simulink library "halin"  (R2021b)
settings: Solver=VariableStepAuto  StartTime=0.0  StopTime=10.0  RelTol=1e-3
undefined symbols (not defined in the file): KHAL_CAN1ABM1E2E_flg, KHAL_CAN1EPB1E2E_flg, KHAL_CAN1EPS1E2E_flg, KHAL_CAN1ESC1E2E_flg, KHAL_CAN1ESC5E2E_flg, KHAL_CAN3BMS1E2E_flg, KHAL_CAN3BMS6E2E_flg, KHAL_CAN3CCU1E2E_flg, KHAL_CAN3CCU2E2E_flg, KHAL_CAN3MCUNF1E2E_flg, KHAL_CAN3MCUNR1E2E_flg, KHAL_CAN3Shifter1E2E_flg, KHAL_CAN3Shifter2E2E_flg, KHAL_CAN6FCM2E2E_flg, KHAL_CAN6FCM4E2E_flg, TRUE
libraries: simulink x645, FVT_lib x207, hcu_lib x59
(part 5 of 23)

== system halin/HAL_IN/CAN5 ==
  DT_CAN5_SG_TBOX1 : Inport
  DT_CAN5_SG_TBOX2 : Inport  Port=2
  DT_CAN5_SG_TBOX3 : Inport  Port=3
  UnitConverter{,2,4,8..10} (6 alike) : DataTypeConversion  OutDataTypeStr=uint8
  UnitConverter{1,6,11..27} (19 alike) : DataTypeConversion  OutDataTypeStr=single
  UnitConverter28 : DataTypeConversion  OutDataTypeStr=uint32
  UnitConverter29 : DataTypeConversion  OutDataTypeStr=uint32
  UnitConverter3 : DataTypeConversion  OutDataTypeStr=uint16
  UnitConverter5 : DataTypeConversion  OutDataTypeStr=boolean
  UnitConverter7 : DataTypeConversion  OutDataTypeStr=boolean
  VHAL_CANMsgInvalidTBOX1_flg : Subsystem  AncestorBlock=FVT_lib/hal/MsgTimeoutJudge_CAN_AUTOSAR
      mask help: MeasumentTrigerEvent
      mask Display: fprintf('MsgTimeoutJudge_CAN\nAUTOSAR');
  VHAL_CANMsgInvalidTBOX2_flg : Subsystem  AncestorBlock=FVT_lib/hal/MsgTimeoutJudge_CAN_AUTOSAR
      mask help: MeasumentTrigerEvent
      mask Display: fprintf('MsgTimeoutJudge_CAN\nAUTOSAR');
  VHAL_CANMsgInvalidTBOX3_flg : Subsystem  AncestorBlock=FVT_lib/hal/MsgTimeoutJudge_CAN_AUTOSAR
      mask help: MeasumentTrigerEvent
      mask Display: fprintf('MsgTimeoutJudge_CAN\nAUTOSAR');
  bus_creator : BusCreator  Inputs=33
  HAL_CAN5_outputs : Outport
  wires:
  DT_CAN5_SG_TBOX1/1 -> [DT_CAN5_SG_TBOX1]
  DT_CAN5_SG_TBOX2/1 -> [DT_CAN5_SG_TBOX2]
  DT_CAN5_SG_TBOX3/1 -> [DT_CAN5_SG_TBOX3]
  bus_creator/1 -> HAL_CAN5_outputs/1
  VHAL_CANMsgInvalidTBOX1_flg/1(Out) -> bus_creator/1
  UnitConverter/1 -> bus_creator/2  "VHAL_CbnPreACEnaReq_enum"
  [VHAL_CbnPreACEnaReq_enum] -> UnitConverter/1
  UnitConverter1/1 -> bus_creator/3  "VHAL_PowerOffTSet_cnt"
  [VHAL_PowerOffTSet_cnt] -> UnitConverter1/1
  UnitConverter2/1 -> bus_creator/4  "VHAL_ReOutsideMirror_enum"
  [VHAL_ReOutsideMirror_enum] -> UnitConverter2/1
  UnitConverter3/1 -> bus_creator/5  "VHAL_ReDoorLock_enum"
  [VHAL_ReDoorLock_enum] -> UnitConverter3/1
  UnitConverter4/1 -> bus_creator/6  "VHAL_RePwrReqTbox_enum"
  [VHAL_RePwrReqTbox_enum] -> UnitConverter4/1
  UnitConverter5/1 -> bus_creator/7  "VHAL_ReRadio_flg"
  [VHAL_ReRadio_flg] -> UnitConverter5/1
  UnitConverter6/1 -> bus_creator/8  "VHAL_RemoteACTemp_C"
  [VHAL_RemoteACTemp_C] -> UnitConverter6/1
  UnitConverter7/1 -> bus_creator/9  "VHAL_RemoteAutoReq_flg"
  [VHAL_RemoteAutoReq_flg] -> UnitConverter7/1
  UnitConverter8/1 -> bus_creator/10  "VHAL_TBOXNETSIGSTR_enum"
  [VHAL_TBOXNETSIGSTR_enum] -> UnitConverter8/1
  UnitConverter9/1 -> bus_creator/11  "VHAL_TBOXRemotePW_enum"
  [VHAL_TBOXRemotePW_enum] -> UnitConverter9/1
  UnitConverter10/1 -> bus_creator/12  "VHAL_TBOXTESTSTATUS_enum"
  [VHAL_TBOXTESTSTATUS_enum] -> UnitConverter10/1
  VHAL_CANMsgInvalidTBOX2_flg/1(Out) -> bus_creator/13
  UnitConverter11/1 -> bus_creator/14  "VHAL_TimeSyncFromBSDay_DAY"
  [VHAL_TimeSyncFromBSDay_DAY] -> UnitConverter11/1
  UnitConverter12/1 -> bus_creator/15  "VHAL_TimeSyncFromBSHour_hr"
  [VHAL_TimeSyncFromBSHour_hr] -> UnitConverter12/1
  UnitConverter13/1 -> bus_creator/16  "VHAL_TimeSyncFromBSMinute_min"
  [VHAL_TimeSyncFromBSMinute_min] -> UnitConverter13/1
  UnitConverter14/1 -> bus_creator/17  "VHAL_TimeSyncFromBSMonth_MONTH"
  [VHAL_TimeSyncFromBSMonth_MONTH] -> UnitConverter14/1
  UnitConverter15/1 -> bus_creator/18  "VHAL_TimeSyncFromBSSecond_s"
  [VHAL_TimeSyncFromBSSecond_s] -> UnitConverter15/1
  UnitConverter16/1 -> bus_creator/19  "VHAL_TimeSyncFromBSYear_YEAR"
  [VHAL_TimeSyncFromBSYear_YEAR] -> UnitConverter16/1
  VHAL_CANMsgInvalidTBOX3_flg/1(Out) -> bus_creator/20
  UnitConverter17/1 -> bus_creator/21  "VHAL_ChargePercentSet_pct"
  [VHAL_ChargePercentSet_pct] -> UnitConverter17/1
  UnitConverter18/1 -> bus_creator/22  "VHAL_ReserveChargeOFFDay_DAY"
  [VHAL_ReserveChargeOFFDay_DAY] -> UnitConverter18/1
  UnitConverter19/1 -> bus_creator/23  "VHAL_ReserveChargeOFFHour_hr"
  [VHAL_ReserveChargeOFFHour_hr] -> UnitConverter19/1
  UnitConverter20/1 -> bus_creator/24  "VHAL_ReserveChargeOFFMinute_min"
  [VHAL_ReserveChargeOFFMinute_min] -> UnitConverter20/1
  UnitConverter21/1 -> bus_creator/25  "VHAL_ReserveChargeOFFMonth_MONTH"
  [VHAL_ReserveChargeOFFMonth_MONTH] -> UnitConverter21/1
  UnitConverter22/1 -> bus_creator/26  "VHAL_ReserveChargeOFFYear_YEAR"
  [VHAL_ReserveChargeOFFYear_YEAR] -> UnitConverter22/1
  UnitConverter23/1 -> bus_creator/27  "VHAL_ReserveChargeOnDay_DAY"
  [VHAL_ReserveChargeOnDay_DAY] -> UnitConverter23/1
  UnitConverter24/1 -> bus_creator/28  "VHAL_ReserveChargeOnHour_hr"
  [VHAL_ReserveChargeOnHour_hr] -> UnitConverter24/1
  UnitConverter25/1 -> bus_creator/29  "VHAL_ReserveChargeOnMinute_min"
  [VHAL_ReserveChargeOnMinute_min] -> UnitConverter25/1
  UnitConverter26/1 -> bus_creator/30  "VHAL_ReserveChargeOnMonth_MONTH"
  [VHAL_ReserveChargeOnMonth_MONTH] -> UnitConverter26/1
  UnitConverter27/1 -> bus_creator/31  "VHAL_ReserveChargeOnYear_YEAR"
  [VHAL_ReserveChargeOnYear_YEAR] -> UnitConverter27/1
  UnitConverter28/1 -> bus_creator/32  "VHAL_TBOXHWVER_enum"
  [VHAL_TBOXHWVER_enum] -> UnitConverter28/1
  UnitConverter29/1 -> bus_creator/33  "VHAL_TBOXSWVER_enum"
  [VHAL_TBOXSWVER_enum] -> UnitConverter29/1

== system halin/HAL_IN/CAN6 ==
  DT_CAN6_SG_FCM1 : Inport
  DT_CAN6_SG_FCM2 : Inport  Port=2
  DT_CAN6_SG_FCM3 : Inport  Port=3
  DT_CAN6_SG_FCM4 : Inport  Port=4
  DT_CAN6_SG_SRR1 : Inport  Port=5
  FCM1 : Subsystem
  FCM2 : Subsystem
  FCM3 : Subsystem
  FCM4 : Subsystem
  SRR1 : Subsystem
  UnitConverter{,1..4,6..7,29..30,44,64..79,82..83,85..86} (30 alike) : DataTypeConversion  OutDataTypeStr=single
  UnitConverter{5,10..14,16,20,22..28,31..35,37..38,41..43,45,47,49,55,59..60,63,88..89,92..93} (36 alike) : DataTypeConversion  OutDataTypeStr=uint8
  UnitConverter{8..9,15,17..19,21,36,39..40,46,48,50..54,56..58,61..62,80..81,84,87,90..91} (28 alike) : DataTypeConversion  OutDataTypeStr=boolean
  VHAL_CANMsgInvalidFCM1_flg : Subsystem  AncestorBlock=FVT_lib/hal/MsgTimeoutJudge_CAN_AUTOSAR
      mask help: MeasumentTrigerEvent
      mask Display: fprintf('MsgTimeoutJudge_CAN\nAUTOSAR');
  VHAL_CANMsgInvalidFCM2_flg : Subsystem  AncestorBlock=FVT_lib/hal/MsgTimeoutJudge_CAN_AUTOSAR
      mask help: MeasumentTrigerEvent
      mask Display: fprintf('MsgTimeoutJudge_CAN\nAUTOSAR');
  VHAL_CANMsgInvalidFCM3_flg : Subsystem  AncestorBlock=FVT_lib/hal/MsgTimeoutJudge_CAN_AUTOSAR
      mask help: MeasumentTrigerEvent
      mask Display: fprintf('MsgTimeoutJudge_CAN\nAUTOSAR');
  VHAL_CANMsgInvalidFCM4_flg : Subsystem  AncestorBlock=FVT_lib/hal/MsgTimeoutJudge_CAN_AUTOSAR
      mask help: MeasumentTrigerEvent
      mask Display: fprintf('MsgTimeoutJudge_CAN\nAUTOSAR');
  VHAL_CANMsgInvalidSRR1_flg : Subsystem  AncestorBlock=FVT_lib/hal/MsgTimeoutJudge_CAN_AUTOSAR
      mask help: MeasumentTrigerEvent
      mask Display: fprintf('MsgTimeoutJudge_CAN\nAUTOSAR');
  bus_creator : BusCreator  Inputs=99
  HAL_CAN6_outputs : Outport
  wires:
  DT_CAN6_SG_FCM1/1 -> [DT_CAN6_SG_FCM1]
  DT_CAN6_SG_FCM2/1 -> [DT_CAN6_SG_FCM2]
  DT_CAN6_SG_FCM3/1 -> [DT_CAN6_SG_FCM3]
  DT_CAN6_SG_FCM4/1 -> [DT_CAN6_SG_FCM4]
  DT_CAN6_SG_SRR1/1 -> [DT_CAN6_SG_SRR1]
  [DT_CAN6_SG_FCM1] -> FCM1/1(DT_CAN6_SG_FCM1)
  [DT_CAN6_SG_FCM2] -> FCM2/1(DT_CAN6_SG_FCM2)
  [DT_CAN6_SG_FCM3] -> FCM3/1(DT_CAN6_SG_FCM3)
  [DT_CAN6_SG_FCM4] -> FCM4/1(DT_CAN6_SG_FCM4)
  [DT_CAN6_SG_SRR1] -> SRR1/1(DT_CAN6_SG_SRR1)
  bus_creator/1 -> HAL_CAN6_outputs/1
  VHAL_CANMsgInvalidFCM1_flg/1(Out) -> bus_creator/1
  FCM1/1(VHAL_ACCComfortBandLower_mps2) -> [VHAL_ACCComfortBandLower_mps2]
  UnitConverter/1 -> bus_creator/2  "VHAL_ACCComfortBandLower_mps2"
  [VHAL_ACCComfortBandLower_mps2] -> UnitConverter/1
  FCM1/2(VHAL_ACCComfortBandUpper_mps2) -> [VHAL_ACCComfortBandUpper_mps2]
  UnitConverter1/1 -> bus_creator/3  "VHAL_ACCComfortBandUpper_mps2"
  [VHAL_ACCComfortBandUpper_mps2] -> UnitConverter1/1
  FCM1/3(VHAL_ACCJerkLowerLimit_mps3) -> [VHAL_ACCJerkLowerLimit_mps3]
  UnitConverter2/1 -> bus_creator/4  "VHAL_ACCJerkLowerLimit_mps3"
  [VHAL_ACCJerkLowerLimit_mps3] -> UnitConverter2/1
  FCM1/4(VHAL_ACCJerkUpperLimit_mps3) -> [VHAL_ACCJerkUpperLimit_mps3]
  UnitConverter3/1 -> bus_creator/5  "VHAL_ACCJerkUpperLimit_mps3"
  [VHAL_ACCJerkUpperLimit_mps3] -> UnitConverter3/1
  FCM1/5(VHAL_ACCObjDist_m) -> [VHAL_ACCObjDist_m]
  UnitConverter4/1 -> bus_creator/6  "VHAL_ACCObjDist_m"
  [VHAL_ACCObjDist_m] -> UnitConverter4/1
  FCM1/6(VHAL_ACCObjDstLvl_enum) -> [VHAL_ACCObjDstLvl_enum]
  UnitConverter5/1 -> bus_creator/7  "VHAL_ACCObjDstLvl_enum"
  [VHAL_ACCObjDstLvl_enum] -> UnitConverter5/1
  FCM1/7(VHAL_ACCObjRelSpd_mps) -> [VHAL_ACCObjRelSpd_mps]
  UnitConverter6/1 -> bus_creator/8  "VHAL_ACCObjRelSpd_mps"
  [VHAL_ACCObjRelSpd_mps] -> UnitConverter6/1
  FCM1/8(VHAL_ACCRequiredAccel_mps2) -> [VHAL_ACCRequiredAccel_mps2]
  UnitConverter7/1 -> bus_creator/9  "VHAL_ACCRequiredAccel_mps2"
  [VHAL_ACCRequiredAccel_mps2] -> UnitConverter7/1
  FCM1/9(VHAL_ACCTakeoverReq_flg) -> [VHAL_ACCTakeoverReq_flg]
  UnitConverter8/1 -> bus_creator/10  "VHAL_ACCTakeoverReq_flg"
  [VHAL_ACCTakeoverReq_flg] -> UnitConverter8/1
  FCM1/10(VHAL_ACCVehHoldReq_flg) -> [VHAL_ACCVehHoldReq_flg]
  UnitConverter9/1 -> bus_creator/11  "VHAL_ACCVehHoldReq_flg"
  [VHAL_ACCVehHoldReq_flg] -> UnitConverter9/1
  FCM1/11(VHAL_ADASACCSta_enum) -> [VHAL_ADASACCSta_enum]
  UnitConverter10/1 -> bus_creator/12  "VHAL_ADASACCSta_enum"
  [VHAL_ADASACCSta_enum] -> UnitConverter10/1
  FCM1/12(VHAL_ADASAEBReq_enum) -> [VHAL_ADASAEBReq_enum]
  UnitConverter11/1 -> bus_creator/13  "VHAL_ADASAEBReq_enum"
  [VHAL_ADASAEBReq_enum] -> UnitConverter11/1
  FCM1/13(VHAL_ADASAEBSta_enum) -> [VHAL_ADASAEBSta_enum]
  UnitConverter12/1 -> bus_creator/14  "VHAL_ADASAEBSta_enum"
  [VHAL_ADASAEBSta_enum] -> UnitConverter12/1
  FCM1/14(VHAL_ADASCAMSpdLim_enum) -> [VHAL_ADASCAMSpdLim_enum]
  UnitConverter13/1 -> bus_creator/15  "VHAL_ADASCAMSpdLim_enum"
  [VHAL_ADASCAMSpdLim_enum] -> UnitConverter13/1
  FCM1/15(VHAL_ADASDBSReq_enum) -> [VHAL_ADASDBSReq_enum]
  UnitConverter14/1 -> bus_creator/16  "VHAL_ADASDBSReq_enum"
  [VHAL_ADASDBSReq_enum] -> UnitConverter14/1
  FCM1/16(VHAL_ADASFCWMute_flg) -> [VHAL_ADASFCWMute_flg]
  UnitConverter15/1 -> bus_creator/17  "VHAL_ADASFCWMute_flg"
  [VHAL_ADASFCWMute_flg] -> UnitConverter15/1
  FCM1/17(VHAL_ADASFCWSta_enum) -> [VHAL_ADASFCWSta_enum]
  UnitConverter16/1 -> bus_creator/18  "VHAL_ADASFCWSta_enum"
  [VHAL_ADASFCWSta_enum] -> UnitConverter16/1
  FCM1/18(VHAL_ADASFaultSta_flg) -> [VHAL_ADASFaultSta_flg]
  UnitConverter17/1 -> bus_creator/19  "VHAL_ADASFaultSta_flg"
  [VHAL_ADASFaultSta_flg] -> UnitConverter17/1
  FCM1/19(VHAL_ADASFltWrnReq_flg) -> [VHAL_ADASFltWrnReq_flg]
  UnitConverter18/1 -> bus_creator/20  "VHAL_ADASFltWrnReq_flg"
  [VHAL_ADASFltWrnReq_flg] -> UnitConverter18/1
  FCM1/20(VHAL_ADASForceIdle_flg) -> [VHAL_ADASForceIdle_flg]
  UnitConverter19/1 -> bus_creator/21  "VHAL_ADASForceIdle_flg"
  [VHAL_ADASForceIdle_flg] -> UnitConverter19/1
  FCM1/21(VHAL_ADASISASta_enum) -> [VHAL_ADASISASta_enum]
  UnitConverter20/1 -> bus_creator/22  "VHAL_ADASISASta_enum"
  [VHAL_ADASISASta_enum] -> UnitConverter20/1
  FCM1/22(VHAL_ADASLDWMute_flg) -> [VHAL_ADASLDWMute_flg]
  UnitConverter21/1 -> bus_creator/23  "VHAL_ADASLDWMute_flg"
  [VHAL_ADASLDWMute_flg] -> UnitConverter21/1
  FCM1/23(VHAL_ADASLDWSta_enum) -> [VHAL_ADASLDWSta_enum]
  UnitConverter22/1 -> bus_creator/24  "VHAL_ADASLDWSta_enum"
  [VHAL_ADASLDWSta_enum] -> UnitConverter22/1
  FCM1/24(VHAL_ADASLFCHandsOffWarning_enum) -> [VHAL_ADASLFCHandsOffWarning_enum]
  UnitConverter23/1 -> bus_creator/25  "VHAL_ADASLFCHandsOffWarning_enum"
  [VHAL_ADASLFCHandsOffWarning_enum] -> UnitConverter23/1
  FCM1/25(VHAL_ADASLFCSta_enum) -> [VHAL_ADASLFCSta_enum]
  UnitConverter24/1 -> bus_creator/26  "VHAL_ADASLFCSta_enum"
  [VHAL_ADASLFCSta_enum] -> UnitConverter24/1
  FCM1/26(VHAL_ADASLFCWarnSound_enum) -> [VHAL_ADASLFCWarnSound_enum]
  UnitConverter25/1 -> bus_creator/27  "VHAL_ADASLFCWarnSound_enum"
  [VHAL_ADASLFCWarnSound_enum] -> UnitConverter25/1
  FCM1/27(VHAL_ADASLKASta_enum) -> [VHAL_ADASLKASta_enum]
  UnitConverter26/1 -> bus_creator/28  "VHAL_ADASLKASta_enum"
  [VHAL_ADASLKASta_enum] -> UnitConverter26/1
  FCM1/28(VHAL_ADASLaneModeL_enum) -> [VHAL_ADASLaneModeL_enum]
  UnitConverter27/1 -> bus_creator/29  "VHAL_ADASLaneModeL_enum"
  [VHAL_ADASLaneModeL_enum] -> UnitConverter27/1
  FCM1/29(VHAL_ADASLaneModeR_enum) -> [VHAL_ADASLaneModeR_enum]
  UnitConverter28/1 -> bus_creator/30  "VHAL_ADASLaneModeR_enum"
  [VHAL_ADASLaneModeR_enum] -> UnitConverter28/1
  FCM1/30(VHAL_ADASLanecurveL_raw32) -> [VHAL_ADASLanecurveL_raw32]
  UnitConverter29/1 -> bus_creator/31  "VHAL_ADASLanecurveL_raw32"
  [VHAL_ADASLanecurveL_raw32] -> UnitConverter29/1
  FCM1/31(VHAL_ADASLanecurveR_raw32) -> [VHAL_ADASLanecurveR_raw32]
  UnitConverter30/1 -> bus_creator/32  "VHAL_ADASLanecurveR_raw32"
  [VHAL_ADASLanecurveR_raw32] -> UnitConverter30/1
  FCM1/32(VHAL_ADASLanetypeL_enum) -> [VHAL_ADASLanetypeL_enum]
  UnitConverter31/1 -> bus_creator/33  "VHAL_ADASLanetypeL_enum"
  [VHAL_ADASLanetypeL_enum] -> UnitConverter31/1
  FCM1/33(VHAL_ADASLanetypeR_enum) -> [VHAL_ADASLanetypeR_enum]
  UnitConverter32/1 -> bus_creator/34  "VHAL_ADASLanetypeR_enum"
  [VHAL_ADASLanetypeR_enum] -> UnitConverter32/1
  FCM1/34(VHAL_ADASSLIFSpdLim_enum) -> [VHAL_ADASSLIFSpdLim_enum]
  UnitConverter33/1 -> bus_creator/35  "VHAL_ADASSLIFSpdLim_enum"
  [VHAL_ADASSLIFSpdLim_enum] -> UnitConverter33/1
  FCM1/35(VHAL_ADASSLIFSta_enum) -> [VHAL_ADASSLIFSta_enum]
  UnitConverter34/1 -> bus_creator/36  "VHAL_ADASSLIFSta_enum"
  [VHAL_ADASSLIFSta_enum] -> UnitConverter34/1
  FCM1/36(VHAL_ADASShftPosnReq_enum) -> [VHAL_ADASShftPosnReq_enum]
  UnitConverter35/1 -> bus_creator/37  "VHAL_ADASShftPosnReq_enum"
  [VHAL_ADASShftPosnReq_enum] -> UnitConverter35/1
  FCM1/37(VHAL_ADASShftPosnReqA_flg) -> [VHAL_ADASShftPosnReqA_flg]
  UnitConverter36/1 -> bus_creator/38  "VHAL_ADASShftPosnReqA_flg"
  [VHAL_ADASShftPosnReqA_flg] -> UnitConverter36/1
  FCM1/38(VHAL_ADASVehSpdLim_enum) -> [VHAL_ADASVehSpdLim_enum]
  UnitConverter37/1 -> bus_creator/39  "VHAL_ADASVehSpdLim_enum"
  [VHAL_ADASVehSpdLim_enum] -> UnitConverter37/1
  FCM1/39(VHAL_ADASWarningMsg_enum) -> [VHAL_ADASWarningMsg_enum]
  UnitConverter38/1 -> bus_creator/40  "VHAL_ADASWarningMsg_enum"
  [VHAL_ADASWarningMsg_enum] -> UnitConverter38/1
  FCM1/40(VHAL_AEBVehHoldReq_flg) -> [VHAL_AEBVehHoldReq_flg]
  UnitConverter39/1 -> bus_creator/41  "VHAL_AEBVehHoldReq_flg"
  [VHAL_AEBVehHoldReq_flg] -> UnitConverter39/1
  FCM1/41(VHAL_CameraBlockage_flg) -> [VHAL_CameraBlockage_flg]
  UnitConverter40/1 -> bus_creator/42  "VHAL_CameraBlockage_flg"
  [VHAL_CameraBlockage_flg] -> UnitConverter40/1
  FCM1/42(VHAL_FCM1Checksum_enum) -> [VHAL_FCM1Checksum_enum]
  UnitConverter41/1 -> bus_creator/43  "VHAL_FCM1Checksum_enum"
  [VHAL_FCM1Checksum_enum] -> UnitConverter41/1
  FCM1/43(VHAL_FCM1LifeCount_enum) -> [VHAL_FCM1LifeCount_enum]
  UnitConverter42/1 -> bus_creator/44  "VHAL_FCM1LifeCount_enum"
  [VHAL_FCM1LifeCount_enum] -> UnitConverter42/1
  FCM1/44(VHAL_FCMACCmode_enum) -> [VHAL_FCMACCmode_enum]
  UnitConverter43/1 -> bus_creator/45  "VHAL_FCMACCmode_enum"
  [VHAL_FCMACCmode_enum] -> UnitConverter43/1
  FCM1/45(VHAL_FCMLKAStrToqReq_Nm) -> [VHAL_FCMLKAStrToqReq_Nm]
  UnitConverter44/1 -> bus_creator/46  "VHAL_FCMLKAStrToqReq_Nm"
  [VHAL_FCMLKAStrToqReq_Nm] -> UnitConverter44/1
  FCM1/46(VHAL_FCMLKATOIAct_enum) -> [VHAL_FCMLKATOIAct_enum]
  UnitConverter45/1 -> bus_creator/47  "VHAL_FCMLKATOIAct_enum"
  [VHAL_FCMLKATOIAct_enum] -> UnitConverter45/1
  FCM1/47(VHAL_FCMLKATOIFault_flg) -> [VHAL_FCMLKATOIFault_flg]
  UnitConverter46/1 -> bus_creator/48  "VHAL_FCMLKATOIFault_flg"
  [VHAL_FCMLKATOIFault_flg] -> UnitConverter46/1
  FCM1/48(VHAL_ForceLowBeam_enum) -> [VHAL_ForceLowBeam_enum]
  UnitConverter47/1 -> bus_creator/49  "VHAL_ForceLowBeam_enum"
  [VHAL_ForceLowBeam_enum] -> UnitConverter47/1
  FCM1/49(VHAL_HazardWarningReq_flg) -> [VHAL_HazardWarningReq_flg]
  UnitConverter48/1 -> bus_creator/50  "VHAL_HazardWarningReq_flg"
  [VHAL_HazardWarningReq_flg] -> UnitConverter48/1
  FCM1/50(VHAL_ISAWarningMsg_enum) -> [VHAL_ISAWarningMsg_enum]
  UnitConverter49/1 -> bus_creator/51  "VHAL_ISAWarningMsg_enum"
  [VHAL_ISAWarningMsg_enum] -> UnitConverter49/1
  FCM1/51(VHAL_LKAHODDisplayWarning_flg) -> [VHAL_LKAHODDisplayWarning_flg]
  UnitConverter50/1 -> bus_creator/52  "VHAL_LKAHODDisplayWarning_flg"
  [VHAL_LKAHODDisplayWarning_flg] -> UnitConverter50/1
  FCM1/52(VHAL_LKAHODSoundWarning_flg) -> [VHAL_LKAHODSoundWarning_flg]
  UnitConverter51/1 -> bus_creator/53  "VHAL_LKAHODSoundWarning_flg"
  [VHAL_LKAHODSoundWarning_flg] -> UnitConverter51/1
  FCM1/53(VHAL_LVDAACCStatusInformation_flg) -> [VHAL_LVDAACCStatusInformation_flg]
  UnitConverter52/1 -> bus_creator/54  "VHAL_LVDAACCStatusInformation_flg"
  [VHAL_LVDAACCStatusInformation_flg] -> UnitConverter52/1
  FCM1/54(VHAL_LVDADisabled_flg) -> [VHAL_LVDADisabled_flg]
  UnitConverter53/1 -> bus_creator/55  "VHAL_LVDADisabled_flg"
  [VHAL_LVDADisabled_flg] -> UnitConverter53/1
  FCM1/55(VHAL_LVDAFailinfo_flg) -> [VHAL_LVDAFailinfo_flg]
  UnitConverter54/1 -> bus_creator/56  "VHAL_LVDAFailinfo_flg"
  [VHAL_LVDAFailinfo_flg] -> UnitConverter54/1
  FCM1/56(VHAL_LVDAMuteSta_enum) -> [VHAL_LVDAMuteSta_enum]
  UnitConverter55/1 -> bus_creator/57  "VHAL_LVDAMuteSta_enum"
  [VHAL_LVDAMuteSta_enum] -> UnitConverter55/1
  FCM1/57(VHAL_LVDAWarning_flg) -> [VHAL_LVDAWarning_flg]
  UnitConverter56/1 -> bus_creator/58  "VHAL_LVDAWarning_flg"
  [VHAL_LVDAWarning_flg] -> UnitConverter56/1
  FCM1/58(VHAL_LeftTurnLightReq_flg) -> [VHAL_LeftTurnLightReq_flg]
  UnitConverter57/1 -> bus_creator/59  "VHAL_LeftTurnLightReq_flg"
  [VHAL_LeftTurnLightReq_flg] -> UnitConverter57/1
  FCM1/59(VHAL_RightTurnLightReq_flg) -> [VHAL_RightTurnLightReq_flg]
  UnitConverter58/1 -> bus_creator/60  "VHAL_RightTurnLightReq_flg"
  [VHAL_RightTurnLightReq_flg] -> UnitConverter58/1
  FCM1/60(VHAL_TargetType_enum) -> [VHAL_TargetType_enum]
  UnitConverter59/1 -> bus_creator/61  "VHAL_TargetType_enum"
  [VHAL_TargetType_enum] -> UnitConverter59/1
  FCM1/61(VHAL_TimeGapLevel_enum) -> [VHAL_TimeGapLevel_enum]
  UnitConverter60/1 -> bus_creator/62  "VHAL_TimeGapLevel_enum"
  [VHAL_TimeGapLevel_enum] -> UnitConverter60/1
  VHAL_CANMsgInvalidFCM2_flg/1(Out) -> bus_creator/63
  FCM2/1(VHAL_FCM2CSErr_flg) -> [VHAL_FCM2CSErr_flg]
  UnitConverter61/1 -> bus_creator/64  "VHAL_FCM2CSErr_flg"
  [VHAL_FCM2CSErr_flg] -> UnitConverter61/1
  FCM2/2(VHAL_FCM2RCErr_flg) -> [VHAL_FCM2RCErr_flg]
  UnitConverter62/1 -> bus_creator/65  "VHAL_FCM2RCErr_flg"
  [VHAL_FCM2RCErr_flg] -> UnitConverter62/1
  FCM2/3(VHAL_ADBVehDst1Val_enum) -> [VHAL_ADBVehDst1Val_enum]
  UnitConverter63/1 -> bus_creator/66  "VHAL_ADBVehDst1Val_enum"
  [VHAL_ADBVehDst1Val_enum] -> UnitConverter63/1
  VHAL_CANMsgInvalidFCM3_flg/1(Out) -> bus_creator/67
  FCM3/1(VHAL_MELaneCurvDervLt_raw32) -> [VHAL_MELaneCurvDervLt_raw32]
  UnitConverter64/1 -> bus_creator/68  "VHAL_MELaneCurvDervLt_raw32"
  [VHAL_MELaneCurvDervLt_raw32] -> UnitConverter64/1
  FCM3/2(VHAL_MELaneCurvDervLt2_raw32) -> [VHAL_MELaneCurvDervLt2_raw32]
  UnitConverter65/1 -> bus_creator/69  "VHAL_MELaneCurvDervLt2_raw32"
  [VHAL_MELaneCurvDervLt2_raw32] -> UnitConverter65/1
  FCM3/3(VHAL_MELaneCurvDervRt_raw32) -> [VHAL_MELaneCurvDervRt_raw32]
  UnitConverter66/1 -> bus_creator/70  "VHAL_MELaneCurvDervRt_raw32"
  [VHAL_MELaneCurvDervRt_raw32] -> UnitConverter66/1
  FCM3/4(VHAL_MELaneCurvDervRt2_raw32) -> [VHAL_MELaneCurvDervRt2_raw32]
  UnitConverter67/1 -> bus_creator/71  "VHAL_MELaneCurvDervRt2_raw32"
  [VHAL_MELaneCurvDervRt2_raw32] -> UnitConverter67/1
  FCM3/5(VHAL_MELaneCurvLt_raw32) -> [VHAL_MELaneCurvLt_raw32]
  UnitConverter68/1 -> bus_creator/72  "VHAL_MELaneCurvLt_raw32"
  [VHAL_MELaneCurvLt_raw32] -> UnitConverter68/1
  FCM3/6(VHAL_MELaneCurvLt2_raw32) -> [VHAL_MELaneCurvLt2_raw32]
  UnitConverter69/1 -> bus_creator/73  "VHAL_MELaneCurvLt2_raw32"
  [VHAL_MELaneCurvLt2_raw32] -> UnitConverter69/1
  FCM3/7(VHAL_MELaneCurvRt_raw32) -> [VHAL_MELaneCurvRt_raw32]
  UnitConverter70/1 -> bus_creator/74  "VHAL_MELaneCurvRt_raw32"
  [VHAL_MELaneCurvRt_raw32] -> UnitConverter70/1
  FCM3/8(VHAL_MELaneCurvRt2_raw32) -> [VHAL_MELaneCurvRt2_raw32]
  UnitConverter71/1 -> bus_creator/75  "VHAL_MELaneCurvRt2_raw32"
  [VHAL_MELaneCurvRt2_raw32] -> UnitConverter71/1
  FCM3/9(VHAL_MELaneHeadAngLt_radians) -> [VHAL_MELaneHeadAngLt_radians]
  UnitConverter72/1 -> bus_creator/76  "VHAL_MELaneHeadAngLt_radians"
  [VHAL_MELaneHeadAngLt_radians] -> UnitConverter72/1
  FCM3/10(VHAL_MELaneHeadAngLt2_radians) -> [VHAL_MELaneHeadAngLt2_radians]
  UnitConverter73/1 -> bus_creator/77  "VHAL_MELaneHeadAngLt2_radians"
  [VHAL_MELaneHeadAngLt2_radians] -> UnitConverter73/1
  FCM3/11(VHAL_MELaneHeadAngRt_radians) -> [VHAL_MELaneHeadAngRt_radians]
  UnitConverter74/1 -> bus_creator/78  "VHAL_MELaneHeadAngRt_radians"
  [VHAL_MELaneHeadAngRt_radians] -> UnitConverter74/1
  FCM3/12(VHAL_MELaneHeadAngRt2_radians) -> [VHAL_MELaneHeadAngRt2_radians]
  UnitConverter75/1 -> bus_creator/79  "VHAL_MELaneHeadAngRt2_radians"
  [VHAL_MELaneHeadAngRt2_radians] -> UnitConverter75/1
  FCM3/13(VHAL_MELanePosLt_m) -> [VHAL_MELanePosLt_m]
  UnitConverter76/1 -> bus_creator/80  "VHAL_MELanePosLt_m"
  [VHAL_MELanePosLt_m] -> UnitConverter76/1
  FCM3/14(VHAL_MELanePosLt2_m) -> [VHAL_MELanePosLt2_m]
  UnitConverter77/1 -> bus_creator/81  "VHAL_MELanePosLt2_m"
  [VHAL_MELanePosLt2_m] -> UnitConverter77/1
  FCM3/15(VHAL_MELanePosRt_m) -> [VHAL_MELanePosRt_m]
  UnitConverter78/1 -> bus_creator/82  "VHAL_MELanePosRt_m"
  [VHAL_MELanePosRt_m] -> UnitConverter78/1
  FCM3/16(VHAL_MELanePosRt2_m) -> [VHAL_MELanePosRt2_m]
  UnitConverter79/1 -> bus_creator/83  "VHAL_MELanePosRt2_m"
  [VHAL_MELanePosRt2_m] -> UnitConverter79/1
  VHAL_CANMsgInvalidFCM4_flg/1(Out) -> bus_creator/84
  FCM4/1(VHAL_FCM4CSErr_flg) -> [VHAL_FCM4CSErr_flg]
  UnitConverter80/1 -> bus_creator/85  "VHAL_FCM4CSErr_flg"
  [VHAL_FCM4CSErr_flg] -> UnitConverter80/1
  FCM4/2(VHAL_FCM4RCErr_flg) -> [VHAL_FCM4RCErr_flg]
  UnitConverter81/1 -> bus_creator/86  "VHAL_FCM4RCErr_flg"
  [VHAL_FCM4RCErr_flg] -> UnitConverter81/1
  FCM4/3(VHAL_ADASAngCtrlTqWeightGain_pct) -> [VHAL_ADASAngCtrlTqWeightGain_pct]
  UnitConverter82/1 -> bus_creator/87  "VHAL_ADASAngCtrlTqWeightGain_pct"
  [VHAL_ADASAngCtrlTqWeightGain_pct] -> UnitConverter82/1
  FCM4/4(VHAL_ADASDesStrWhlAngCtrlCmd_Deg) -> [VHAL_ADASDesStrWhlAngCtrlCmd_Deg]
  UnitConverter83/1 -> bus_creator/88  "VHAL_ADASDesStrWhlAngCtrlCmd_Deg"
  [VHAL_ADASDesStrWhlAngCtrlCmd_Deg] -> UnitConverter83/1
  FCM4/5(VHAL_ADASDrvInputTqBoostAct_flg) -> [VHAL_ADASDrvInputTqBoostAct_flg]
  UnitConverter84/1 -> bus_creator/89  "VHAL_ADASDrvInputTqBoostAct_flg"
  [VHAL_ADASDrvInputTqBoostAct_flg] -> UnitConverter84/1
  FCM4/6(VHAL_ADASDrvInputTqBoostGain_pct) -> [VHAL_ADASDrvInputTqBoostGain_pct]
  UnitConverter85/1 -> bus_creator/90  "VHAL_ADASDrvInputTqBoostGain_pct"
  [VHAL_ADASDrvInputTqBoostGain_pct] -> UnitConverter85/1
  FCM4/7(VHAL_ADASMaxAngCtrlOutTqLimit_Nm) -> [VHAL_ADASMaxAngCtrlOutTqLimit_Nm]
  UnitConverter86/1 -> bus_creator/91  "VHAL_ADASMaxAngCtrlOutTqLimit_Nm"
  [VHAL_ADASMaxAngCtrlOutTqLimit_Nm] -> UnitConverter86/1
  FCM4/8(VHAL_ADASStrWhlAngCtrlStatus_flg) -> [VHAL_ADASStrWhlAngCtrlStatus_flg]
  UnitConverter87/1 -> bus_creator/92  "VHAL_ADASStrWhlAngCtrlStatus_flg"
  [VHAL_ADASStrWhlAngCtrlStatus_flg] -> UnitConverter87/1
  VHAL_CANMsgInvalidSRR1_flg/1(Out) -> bus_creator/93
  SRR1/1(VHAL_SRRBSDWarnL_enum) -> [VHAL_SRRBSDWarnL_enum]
  UnitConverter88/1 -> bus_creator/94  "VHAL_SRRBSDWarnL_enum"
  [VHAL_SRRBSDWarnL_enum] -> UnitConverter88/1
  SRR1/2(VHAL_SRRBSDWarnR_enum) -> [VHAL_SRRBSDWarnR_enum]
  UnitConverter89/1 -> bus_creator/95  "VHAL_SRRBSDWarnR_enum"
  [VHAL_SRRBSDWarnR_enum] -> UnitConverter89/1
  SRR1/3(VHAL_SRRODASoundL_flg) -> [VHAL_SRRODASoundL_flg]
  UnitConverter90/1 -> bus_creator/96  "VHAL_SRRODASoundL_flg"
  [VHAL_SRRODASoundL_flg] -> UnitConverter90/1
  SRR1/4(VHAL_SRRODASoundR_flg) -> [VHAL_SRRODASoundR_flg]
  UnitConverter91/1 -> bus_creator/97  "VHAL_SRRODASoundR_flg"
  [VHAL_SRRODASoundR_flg] -> UnitConverter91/1
  SRR1/5(VHAL_SRRODAWarnL_enum) -> [VHAL_SRRODAWarnL_enum]
  UnitConverter92/1 -> bus_creator/98  "VHAL_SRRODAWarnL_enum"
  [VHAL_SRRODAWarnL_enum] -> UnitConverter92/1
  SRR1/6(VHAL_SRRODAWarnR_enum) -> [VHAL_SRRODAWarnR_enum]
  UnitConverter93/1 -> bus_creator/99  "VHAL_SRRODAWarnR_enum"
  [VHAL_SRRODAWarnR_enum] -> UnitConverter93/1

== system halin/HAL_IN/CAN1/ABM1 ==
  DT_CAN1_SG_ABM1 : Inport
  0xE4 : Constant  Value=0xE4
  0xF2 : Constant  Value=0xF2
  ABMPassengerODSSta : Subsystem
  ABMRearPassengerCTRODSSta : Subsystem
  ABMRearPassengerLHODSSta : Subsystem
  ABMRearPassengerRHODSSta : Subsystem
  AirBagFailCmd : Subsystem
  BitwiseAND{,1..15} (16 alike) : simulink/Logic and Bit Operations/Bitwise Operator  logicop=AND  UseBitMask=on  BitMask=0xFF  BitMaskRealWorld=Stored Integer
  BitwiseOR : simulink/Logic and Bit Operations/Bitwise Operator  logicop=OR  UseBitMask=off  BitMask=bin2dec('11011001')  BitMaskRealWorld=Stored Integer
  BitwiseOR1 : simulink/Logic and Bit Operations/Bitwise Operator  logicop=OR  UseBitMask=off  BitMask=bin2dec('11011001')  BitMaskRealWorld=Stored Integer
  BitwiseOR2 : simulink/Logic and Bit Operations/Bitwise Operator  logicop=OR  UseBitMask=off  BitMask=bin2dec('11011001')  BitMaskRealWorld=Stored Integer
  BitwiseOR3 : simulink/Logic and Bit Operations/Bitwise Operator  logicop=OR  UseBitMask=off  NumInputPorts=5  BitMask=bin2dec('11011001')  BitMaskRealWorld=Stored Integer
  BitwiseOR4 : simulink/Logic and Bit Operations/Bitwise Operator  logicop=OR  UseBitMask=off  NumInputPorts=8  BitMask=bin2dec('11011001')  BitMaskRealWorld=Stored Integer
  ChecksumABM1 : Subsystem
  CrashOutputSts : Subsystem
  DDM_CS&RC_Comparison : FVT_lib/hal/DDM_CS&RC_Comparison  MsgCycleTime=500
  Data Type Conversion{,1..15} (16 alike) : DataTypeConversion  OutDataTypeStr=uint8
  DriverSeatBeltCmd : Subsystem
  KHAL_CAN1ABM1E2E_flg : Constant  Value=KHAL_CAN1ABM1E2E_flg
  LeftShift : ArithShift  BitShiftNumber=4  BitShiftDirection=Left
  LeftShift1 : ArithShift  BitShiftNumber=2  BitShiftDirection=Left
  LeftShift10 : ArithShift  BitShiftNumber=2  BitShiftDirection=Left
  LeftShift11 : ArithShift  BitShiftNumber=6  BitShiftDirection=Left
  LeftShift12 : ArithShift  BitShiftNumber=4  BitShiftDirection=Left
  LeftShift13 : ArithShift  BitShiftNumber=5  BitShiftDirection=Left
  LeftShift14 : ArithShift  BitShiftNumber=7  BitShiftDirection=Left
  LeftShift{4..6,8,15} (5 alike) : ArithShift  BitShiftDirection=Left
  LeftShift2 : ArithShift  BitShiftNumber=3  BitShiftDirection=Left
  LeftShift3 : ArithShift  BitShiftNumber=1  BitShiftDirection=Left
  LeftShift7 : ArithShift  BitShiftNumber=1  BitShiftDirection=Left
  LeftShift9 : ArithShift  BitShiftNumber=3  BitShiftDirection=Left
  LifeCountABM1 : Subsystem
  MessageRollingCounter : FVT_lib/hal/MessageRollingCounter  CounterMAX=14  task_time_ms=5  msg_time_ms=500
  Mux : Mux  Inputs=7
  PABSwitchCmd : Subsystem
  PsngrSeatBeltCmd : Subsystem
  RCenterSeatBeltCmd : Subsystem
  RDriverSeatBeltCmd : Subsystem
  RPsngrSeatBeltCmd : Subsystem
  TLHPsngrSeatBeltCmd : Subsystem
  TRHPsngrSeatBeltCmd : Subsystem
  bus_selector : BusSelector  OutputSignals=CAN1_ABM_Passenger_ODS_Sta,CAN1_ABM_RearPassengerCTR_ODS_Sta,CAN1_ABM_RearPassengerLH_ODS_Sta,CAN1_ABM_RearPassengerRH_ODS_Sta,CAN1_AirBagFailCmd,CAN1_Checksum_ABM1,CAN1_CrashOutputSts,CAN1_DriverSeatBeltCmd,CAN1_LifeCount_ABM1,CAN1_PABSwitchCmd,CAN1_PsngrSeatBeltCmd,CAN1_RCenterSeatBeltCmd,CAN1_RDriverSeatBeltCmd,CAN1_RPsngrSeatBeltCmd,CAN1_TLHPsngrSeatBeltCmd,CAN1_TRHPsngrSeatBeltCmd
  bus_selector1 : BusSelector  OutputSignals=CAN1_ABM_Passenger_ODS_Sta
  bus_selector10 : BusSelector  OutputSignals=CAN1_PABSwitchCmd
  bus_selector11 : BusSelector  OutputSignals=CAN1_PsngrSeatBeltCmd
  bus_selector12 : BusSelector  OutputSignals=CAN1_RCenterSeatBeltCmd
  bus_selector13 : BusSelector  OutputSignals=CAN1_RDriverSeatBeltCmd
  bus_selector14 : BusSelector  OutputSignals=CAN1_RPsngrSeatBeltCmd
  bus_selector15 : BusSelector  OutputSignals=CAN1_TLHPsngrSeatBeltCmd
  bus_selector16 : BusSelector  OutputSignals=CAN1_TRHPsngrSeatBeltCmd
  bus_selector2 : BusSelector  OutputSignals=CAN1_ABM_RearPassengerCTR_ODS_Sta
  bus_selector3 : BusSelector  OutputSignals=CAN1_ABM_RearPassengerLH_ODS_Sta
  bus_selector4 : BusSelector  OutputSignals=CAN1_ABM_RearPassengerRH_ODS_Sta
  bus_selector5 : BusSelector  OutputSignals=CAN1_AirBagFailCmd
  bus_selector6 : BusSelector  OutputSignals=CAN1_Checksum_ABM1
  bus_selector7 : BusSelector  OutputSignals=CAN1_CrashOutputSts
  bus_selector8 : BusSelector  OutputSignals=CAN1_DriverSeatBeltCmd
  bus_selector9 : BusSelector  OutputSignals=CAN1_LifeCount_ABM1
  constant : Constant  Value=0x0  OutDataTypeStr=uint8
  constant1 : Constant  Value=0x0  OutDataTypeStr=uint8
  constant2 : Constant  Value=0x0  OutDataTypeStr=uint8
  VHAL_ABM1CSErr_flg : Outport
  VHAL_ABM1RCErr_flg : Outport  Port=2
  VHAL_ABMPassengerODSSta_flg : Outport  Port=3
  VHAL_ABMRearPassengerCTRODSSta_flg : Outport  Port=4
  VHAL_ABMRearPassengerLHODSSta_flg : Outport  Port=5
  VHAL_ABMRearPassengerRHODSSta_flg : Outport  Port=6
  VHAL_AirBagFailCmd_flg : Outport  Port=7
  VHAL_ChecksumABM1_enum : Outport  Port=8
  VHAL_CrashOutputSts_enum : Outport  Port=9
  VHAL_DriverSeatBeltCmd_flg : Outport  Port=10
  VHAL_LifeCountABM1_enum : Outport  Port=11
  VHAL_PABSwitchCmd_flg : Outport  Port=12
  VHAL_PsngrSeatBeltCmd_flg : Outport  Port=13
  VHAL_RCenterSeatBeltCmd_flg : Outport  Port=14
  VHAL_RDriverSeatBeltCmd_flg : Outport  Port=15
  VHAL_RPsngrSeatBeltCmd_flg : Outport  Port=16
  VHAL_TLHPsngrSeatBeltCmd_flg : Outport  Port=17
  VHAL_TRHPsngrSeatBeltCmd_flg : Outport  Port=18
  wires:
  DT_CAN1_SG_ABM1/1 -> [DT_CAN1_SG_ABM1]
  [DT_CAN1_SG_ABM1] -> bus_selector/1
  bus_selector/1 -> [CAN1_ABM_Passenger_ODS_Sta]  "<CAN1_ABM_Passenger_ODS_Sta>"
  [CAN1_ABM_Passenger_ODS_Sta] -> LeftShift/1
  LeftShift/1 -> BitwiseAND/1
  BitwiseAND/1 -> [Byte_6_CAN1_ABM_Passenger_ODS_Sta]
  bus_selector/2 -> [CAN1_ABM_RearPassengerCTR_ODS_Sta]  "<CAN1_ABM_RearPassengerCTR_ODS_Sta>"
  [CAN1_ABM_RearPassengerCTR_ODS_Sta] -> LeftShift1/1
  LeftShift1/1 -> BitwiseAND1/1
  BitwiseAND1/1 -> [Byte_6_CAN1_ABM_RearPassengerCTR_ODS_Sta]
  bus_selector/3 -> [CAN1_ABM_RearPassengerLH_ODS_Sta]  "<CAN1_ABM_RearPassengerLH_ODS_Sta>"
  [CAN1_ABM_RearPassengerLH_ODS_Sta] -> LeftShift2/1
  LeftShift2/1 -> BitwiseAND2/1
  BitwiseAND2/1 -> [Byte_6_CAN1_ABM_RearPassengerLH_ODS_Sta]
  bus_selector/4 -> [CAN1_ABM_RearPassengerRH_ODS_Sta]  "<CAN1_ABM_RearPassengerRH_ODS_Sta>"
  [CAN1_ABM_RearPassengerRH_ODS_Sta] -> LeftShift3/1
  LeftShift3/1 -> BitwiseAND3/1
  BitwiseAND3/1 -> [Byte_6_CAN1_ABM_RearPassengerRH_ODS_Sta]
  bus_selector/5 -> [CAN1_AirBagFailCmd]  "<CAN1_AirBagFailCmd>"
  [CAN1_AirBagFailCmd] -> LeftShift4/1
  LeftShift4/1 -> BitwiseAND4/1
  BitwiseAND4/1 -> [Byte_7_CAN1_AirBagFailCmd]
  bus_selector/6 -> [CAN1_Checksum_ABM1]  "<CAN1_Checksum_ABM1>"
  [CAN1_Checksum_ABM1] -> LeftShift5/1
  LeftShift5/1 -> BitwiseAND5/1
  BitwiseAND5/1 -> [Byte_0_CAN1_Checksum_ABM1]
  bus_selector/7 -> [CAN1_CrashOutputSts]  "<CAN1_CrashOutputSts>"
  [CAN1_CrashOutputSts] -> LeftShift6/1
  LeftShift6/1 -> BitwiseAND6/1
  BitwiseAND6/1 -> [Byte_5_CAN1_CrashOutputSts]
  bus_selector/8 -> [CAN1_DriverSeatBeltCmd]  "<CAN1_DriverSeatBeltCmd>"
  [CAN1_DriverSeatBeltCmd] -> LeftShift7/1
  LeftShift7/1 -> BitwiseAND7/1
  BitwiseAND7/1 -> [Byte_7_CAN1_DriverSeatBeltCmd]
  bus_selector/9 -> [CAN1_LifeCount_ABM1]  "<CAN1_LifeCount_ABM1>"
  [CAN1_LifeCount_ABM1] -> LeftShift8/1
  LeftShift8/1 -> BitwiseAND8/1
  BitwiseAND8/1 -> [Byte_1_CAN1_LifeCount_ABM1]
  bus_selector/10 -> [CAN1_PABSwitchCmd]  "<CAN1_PABSwitchCmd>"
  [CAN1_PABSwitchCmd] -> LeftShift9/1
  LeftShift9/1 -> BitwiseAND9/1
  BitwiseAND9/1 -> [Byte_7_CAN1_PABSwitchCmd]
  bus_selector/11 -> [CAN1_PsngrSeatBeltCmd]  "<CAN1_PsngrSeatBeltCmd>"
  [CAN1_PsngrSeatBeltCmd] -> LeftShift10/1
  LeftShift10/1 -> BitwiseAND10/1
  BitwiseAND10/1 -> [Byte_7_CAN1_PsngrSeatBeltCmd]
  bus_selector/12 -> [CAN1_RCenterSeatBeltCmd]  "<CAN1_RCenterSeatBeltCmd>"
  [CAN1_RCenterSeatBeltCmd] -> LeftShift11/1
  LeftShift11/1 -> BitwiseAND11/1
  BitwiseAND11/1 -> [Byte_7_CAN1_RCenterSeatBeltCmd]
  bus_selector/13 -> [CAN1_RDriverSeatBeltCmd]  "<CAN1_RDriverSeatBeltCmd>"
  [CAN1_RDriverSeatBeltCmd] -> LeftShift12/1
  LeftShift12/1 -> BitwiseAND12/1
  BitwiseAND12/1 -> [Byte_7_CAN1_RDriverSeatBeltCmd]
  bus_selector/14 -> [CAN1_RPsngrSeatBeltCmd]  "<CAN1_RPsngrSeatBeltCmd>"
  [CAN1_RPsngrSeatBeltCmd] -> LeftShift13/1
  LeftShift13/1 -> BitwiseAND13/1
  BitwiseAND13/1 -> [Byte_7_CAN1_RPsngrSeatBeltCmd]
  bus_selector/15 -> [CAN1_TLHPsngrSeatBeltCmd]  "<CAN1_TLHPsngrSeatBeltCmd>"
  [CAN1_TLHPsngrSeatBeltCmd] -> LeftShift14/1
  LeftShift14/1 -> BitwiseAND14/1
  BitwiseAND14/1 -> [Byte_7_CAN1_TLHPsngrSeatBeltCmd]
  bus_selector/16 -> [CAN1_TRHPsngrSeatBeltCmd]  "<CAN1_TRHPsngrSeatBeltCmd>"
  [CAN1_TRHPsngrSeatBeltCmd] -> LeftShift15/1
  LeftShift15/1 -> BitwiseAND15/1
  BitwiseAND15/1 -> [Byte_6_CAN1_TRHPsngrSeatBeltCmd]
  Data Type Conversion/1 -> BitwiseOR/1
  [Byte_0_CAN1_Checksum_ABM1] -> Data Type Conversion/1
  BitwiseOR/1 -> [Byte_0]
  Data Type Conversion1/1 -> BitwiseOR1/1
  [Byte_1_CAN1_LifeCount_ABM1] -> Data Type Conversion1/1
  BitwiseOR1/1 -> [Byte_1]
  constant/1 -> [Byte_2]
  constant1/1 -> [Byte_3]
  constant2/1 -> [Byte_4]
  Data Type Conversion2/1 -> BitwiseOR2/1
  [Byte_5_CAN1_CrashOutputSts] -> Data Type Conversion2/1
  BitwiseOR2/1 -> [Byte_5]
  Data Type Conversion3/1 -> BitwiseOR3/1
  [Byte_6_CAN1_ABM_Passenger_ODS_Sta] -> Data Type Conversion3/1
  Data Type Conversion4/1 -> BitwiseOR3/2
  [Byte_6_CAN1_ABM_RearPassengerCTR_ODS_Sta] -> Data Type Conversion4/1
  Data Type Conversion5/1 -> BitwiseOR3/3
  [Byte_6_CAN1_ABM_RearPassengerLH_ODS_Sta] -> Data Type Conversion5/1
  Data Type Conversion6/1 -> BitwiseOR3/4
  [Byte_6_CAN1_ABM_RearPassengerRH_ODS_Sta] -> Data Type Conversion6/1
  Data Type Conversion7/1 -> BitwiseOR3/5
  [Byte_6_CAN1_TRHPsngrSeatBeltCmd] -> Data Type Conversion7/1
  BitwiseOR3/1 -> [Byte_6]
  Data Type Conversion8/1 -> BitwiseOR4/1
  [Byte_7_CAN1_AirBagFailCmd] -> Data Type Conversion8/1
  Data Type Conversion9/1 -> BitwiseOR4/2
  [Byte_7_CAN1_DriverSeatBeltCmd] -> Data Type Conversion9/1
  Data Type Conversion10/1 -> BitwiseOR4/3
  [Byte_7_CAN1_PABSwitchCmd] -> Data Type Conversion10/1
  Data Type Conversion11/1 -> BitwiseOR4/4
  [Byte_7_CAN1_PsngrSeatBeltCmd] -> Data Type Conversion11/1
  Data Type Conversion12/1 -> BitwiseOR4/5
  [Byte_7_CAN1_RCenterSeatBeltCmd] -> Data Type Conversion12/1
  Data Type Conversion13/1 -> BitwiseOR4/6
  [Byte_7_CAN1_RDriverSeatBeltCmd] -> Data Type Conversion13/1
  Data Type Conversion14/1 -> BitwiseOR4/7
  [Byte_7_CAN1_RPsngrSeatBeltCmd] -> Data Type Conversion14/1
  Data Type Conversion15/1 -> BitwiseOR4/8
  [Byte_7_CAN1_TLHPsngrSeatBeltCmd] -> Data Type Conversion15/1
  BitwiseOR4/1 -> [Byte_7]
  [Byte_1] -> Mux/1
  [Byte_2] -> Mux/2
  [Byte_3] -> Mux/3
  [Byte_4] -> Mux/4
  [Byte_5] -> Mux/5
  [Byte_6] -> Mux/6
  [Byte_7] -> Mux/7
  Mux/1 -> [VHAL_CAN1ABM1noCS_raw]
  KHAL_CAN1ABM1E2E_flg/1 -> DDM_CS&RC_Comparison/1
  0xF2/1 -> DDM_CS&RC_Comparison/2
  0xE4/1 -> DDM_CS&RC_Comparison/3
  [VHAL_CAN1ABM1noCS_raw] -> DDM_CS&RC_Comparison/4
  [Byte_0] -> DDM_CS&RC_Comparison/5
  [RC_ECU] -> DDM_CS&RC_Comparison/6
  MessageRollingCounter/1 -> DDM_CS&RC_Comparison/7
  DDM_CS&RC_Comparison/1 -> VHAL_ABM1CSErr_flg/1
  DDM_CS&RC_Comparison/2 -> VHAL_ABM1RCErr_flg/1
  [DT_CAN1_SG_ABM1] -> bus_selector1/1
  bus_selector1/1 -> ABMPassengerODSSta/1(ABM_Passenger_ODS_Sta)  "<CAN1_ABM_Passenger_ODS_Sta>"
  ABMPassengerODSSta/1(VHAL_ABMPassengerODSSta_flg) -> VHAL_ABMPassengerODSSta_flg/1
  [DT_CAN1_SG_ABM1] -> bus_selector2/1
  bus_selector2/1 -> ABMRearPassengerCTRODSSta/1(ABM_RearPassengerCTR_ODS_Sta)  "<CAN1_ABM_RearPassengerCTR_ODS_Sta>"
  ABMRearPassengerCTRODSSta/1(VHAL_ABMRearPassengerCTRODSSta_flg) -> VHAL_ABMRearPassengerCTRODSSta_flg/1
  [DT_CAN1_SG_ABM1] -> bus_selector3/1
  bus_selector3/1 -> ABMRearPassengerLHODSSta/1(ABM_RearPassengerLH_ODS_Sta)  "<CAN1_ABM_RearPassengerLH_ODS_Sta>"
  ABMRearPassengerLHODSSta/1(VHAL_ABMRearPassengerLHODSSta_flg) -> VHAL_ABMRearPassengerLHODSSta_flg/1
  [DT_CAN1_SG_ABM1] -> bus_selector4/1
  bus_selector4/1 -> ABMRearPassengerRHODSSta/1(ABM_RearPassengerRH_ODS_Sta)  "<CAN1_ABM_RearPassengerRH_ODS_Sta>"
  ABMRearPassengerRHODSSta/1(VHAL_ABMRearPassengerRHODSSta_flg) -> VHAL_ABMRearPassengerRHODSSta_flg/1
  [DT_CAN1_SG_ABM1] -> bus_selector5/1
  bus_selector5/1 -> AirBagFailCmd/1(AirBagFailCmd)  "<CAN1_AirBagFailCmd>"
  AirBagFailCmd/1(VHAL_AirBagFailCmd_flg) -> VHAL_AirBagFailCmd_flg/1
  [DT_CAN1_SG_ABM1] -> bus_selector6/1
  bus_selector6/1 -> ChecksumABM1/1(Checksum_ABM1)  "<CAN1_Checksum_ABM1>"
  ChecksumABM1/1(VHAL_ChecksumABM1_enum) -> VHAL_ChecksumABM1_enum/1
  [DT_CAN1_SG_ABM1] -> bus_selector7/1
  bus_selector7/1 -> CrashOutputSts/1(CrashOutputSts)  "<CAN1_CrashOutputSts>"
  CrashOutputSts/1(VHAL_CrashOutputSts_enum) -> VHAL_CrashOutputSts_enum/1
  [DT_CAN1_SG_ABM1] -> bus_selector8/1
  bus_selector8/1 -> DriverSeatBeltCmd/1(DriverSeatBeltCmd)  "<CAN1_DriverSeatBeltCmd>"
  DriverSeatBeltCmd/1(VHAL_DriverSeatBeltCmd_flg) -> VHAL_DriverSeatBeltCmd_flg/1
  [DT_CAN1_SG_ABM1] -> bus_selector9/1
  bus_selector9/1 -> LifeCountABM1/1(LifeCount_ABM1)  "<CAN1_LifeCount_ABM1>"
  LifeCountABM1/1(VHAL_LifeCountABM1_enum) -> VHAL_LifeCountABM1_enum/1, [RC_ECU]
  [DT_CAN1_SG_ABM1] -> bus_selector10/1
  bus_selector10/1 -> PABSwitchCmd/1(PABSwitchCmd)  "<CAN1_PABSwitchCmd>"
  PABSwitchCmd/1(VHAL_PABSwitchCmd_flg) -> VHAL_PABSwitchCmd_flg/1
  [DT_CAN1_SG_ABM1] -> bus_selector11/1
  bus_selector11/1 -> PsngrSeatBeltCmd/1(PsngrSeatBeltCmd)  "<CAN1_PsngrSeatBeltCmd>"
  PsngrSeatBeltCmd/1(VHAL_PsngrSeatBeltCmd_flg) -> VHAL_PsngrSeatBeltCmd_flg/1
  [DT_CAN1_SG_ABM1] -> bus_selector12/1
  bus_selector12/1 -> RCenterSeatBeltCmd/1(RCenterSeatBeltCmd)  "<CAN1_RCenterSeatBeltCmd>"
  RCenterSeatBeltCmd/1(VHAL_RCenterSeatBeltCmd_flg) -> VHAL_RCenterSeatBeltCmd_flg/1
  [DT_CAN1_SG_ABM1] -> bus_selector13/1
  bus_selector13/1 -> RDriverSeatBeltCmd/1(RDriverSeatBeltCmd)  "<CAN1_RDriverSeatBeltCmd>"
  RDriverSeatBeltCmd/1(VHAL_RDriverSeatBeltCmd_flg) -> VHAL_RDriverSeatBeltCmd_flg/1
  [DT_CAN1_SG_ABM1] -> bus_selector14/1
  bus_selector14/1 -> RPsngrSeatBeltCmd/1(RPsngrSeatBeltCmd)  "<CAN1_RPsngrSeatBeltCmd>"
  RPsngrSeatBeltCmd/1(VHAL_RPsngrSeatBeltCmd_flg) -> VHAL_RPsngrSeatBeltCmd_flg/1
  [DT_CAN1_SG_ABM1] -> bus_selector15/1
  bus_selector15/1 -> TLHPsngrSeatBeltCmd/1(TLHPsngrSeatBeltCmd)  "<CAN1_TLHPsngrSeatBeltCmd>"
  TLHPsngrSeatBeltCmd/1(VHAL_TLHPsngrSeatBeltCmd_flg) -> VHAL_TLHPsngrSeatBeltCmd_flg/1
  [DT_CAN1_SG_ABM1] -> bus_selector16/1
  bus_selector16/1 -> TRHPsngrSeatBeltCmd/1(TRHPsngrSeatBeltCmd)  "<CAN1_TRHPsngrSeatBeltCmd>"
  TRHPsngrSeatBeltCmd/1(VHAL_TRHPsngrSeatBeltCmd_flg) -> VHAL_TRHPsngrSeatBeltCmd_flg/1

== system halin/HAL_IN/CAN1/EPB1 ==
  DT_CAN1_SG_EPB1 : Inport
  0x2B : Constant  Value=0x2B
  0x7A : Constant  Value=0x7A
  BitwiseAND{,1..12} (13 alike) : simulink/Logic and Bit Operations/Bitwise Operator  logicop=AND  UseBitMask=on  BitMask=0xFF  BitMaskRealWorld=Stored Integer
  BitwiseOR : simulink/Logic and Bit Operations/Bitwise Operator  logicop=OR  UseBitMask=off  BitMask=bin2dec('11011001')  BitMaskRealWorld=Stored Integer
  BitwiseOR1 : simulink/Logic and Bit Operations/Bitwise Operator  logicop=OR  UseBitMask=off  BitMask=bin2dec('11011001')  BitMaskRealWorld=Stored Integer
  BitwiseOR2 : simulink/Logic and Bit Operations/Bitwise Operator  logicop=OR  UseBitMask=off  NumInputPorts=2  BitMask=bin2dec('11011001')  BitMaskRealWorld=Stored Integer
  BitwiseOR3 : simulink/Logic and Bit Operations/Bitwise Operator  logicop=OR  UseBitMask=off  NumInputPorts=3  BitMask=bin2dec('11011001')  BitMaskRealWorld=Stored Integer
  BitwiseOR4 : simulink/Logic and Bit Operations/Bitwise Operator  logicop=OR  UseBitMask=off  NumInputPorts=6  BitMask=bin2dec('11011001')  BitMaskRealWorld=Stored Integer
  DDM_CS&RC_Comparison : FVT_lib/hal/DDM_CS&RC_Comparison  MsgCycleTime=40
  DOASta : Subsystem
  Data Type Conversion{,1..12} (13 alike) : DataTypeConversion  OutDataTypeStr=uint8
  EPB1RC : Subsystem
  EPBCarWashMode : Subsystem
  EPBErrSta : Subsystem
  EPBExtApplyAvail : Subsystem
  EPBExtReleaseAvail : Subsystem
  EPBSta : Subsystem
  KHAL_CAN1EPB1E2E_flg : Constant  Value=KHAL_CAN1EPB1E2E_flg
  LeftShift : ArithShift  BitShiftNumber=3  BitShiftDirection=Left
  LeftShift{1..2,6,9,11} (5 alike) : ArithShift  BitShiftDirection=Left
  LeftShift10 : ArithShift  BitShiftNumber=4  BitShiftDirection=Left
  LeftShift12 : ArithShift  BitShiftNumber=7  BitShiftDirection=Left
  LeftShift3 : ArithShift  BitShiftNumber=2  BitShiftDirection=Left
  LeftShift4 : ArithShift  BitShiftNumber=4  BitShiftDirection=Left
  LeftShift5 : ArithShift  BitShiftNumber=1  BitShiftDirection=Left
  LeftShift7 : ArithShift  BitShiftNumber=4  BitShiftDirection=Left
  LeftShift8 : ArithShift  BitShiftNumber=6  BitShiftDirection=Left
  MessageRollingCounter : FVT_lib/hal/MessageRollingCounter  CounterMAX=14  task_time_ms=5  msg_time_ms=40
  Mux : Mux  Inputs=7
  bus_selector : BusSelector  OutputSignals=CAN1_DOA_Sta,CAN1_EPB1_CS,CAN1_EPB1_RC,CAN1_EPBCarWashMode,CAN1_EPBErrSta,CAN1_EPBExtApplyAvail,CAN1_EPBExtReleaseAvail,CAN1_EPBMsg,CAN1_EPBRLampSta,CAN1_EPBSta,CAN1_EPBStaL,CAN1_EPBStaR,CAN1_TakeOverReq
  bus_selector1 : BusSelector  OutputSignals=CAN1_DOA_Sta
  bus_selector2 : BusSelector  OutputSignals=CAN1_EPB1_RC
  bus_selector3 : BusSelector  OutputSignals=CAN1_EPBCarWashMode
  bus_selector4 : BusSelector  OutputSignals=CAN1_EPBErrSta
  bus_selector5 : BusSelector  OutputSignals=CAN1_EPBExtApplyAvail
  bus_selector6 : BusSelector  OutputSignals=CAN1_EPBExtReleaseAvail
  bus_selector7 : BusSelector  OutputSignals=CAN1_EPBSta
  constant : Constant  Value=0x0  OutDataTypeStr=uint8
  constant1 : Constant  Value=0x0  OutDataTypeStr=uint8
  constant2 : Constant  Value=0x0  OutDataTypeStr=uint8
  VHAL_EPB1CSErr_flg : Outport
  VHAL_EPB1RCErr_flg : Outport  Port=2
  VHAL_DOASta_flg : Outport  Port=3
  VHAL_EPB1RC_enum : Outport  Port=4
  VHAL_EPBCarWashMode_flg : Outport  Port=5
  VHAL_EPBErrSta_enum : Outport  Port=6
  VHAL_EPBExtApplyAvail_flg : Outport  Port=7
  VHAL_EPBExtReleaseAvail_flg : Outport  Port=8
  VHAL_EPBSta_enum : Outport  Port=9
  wires:
  DT_CAN1_SG_EPB1/1 -> [DT_CAN1_SG_EPB1]
  [DT_CAN1_SG_EPB1] -> bus_selector/1
  bus_selector/1 -> [CAN1_DOA_Sta]  "<CAN1_DOA_Sta>"
  [CAN1_DOA_Sta] -> LeftShift/1
  LeftShift/1 -> BitwiseAND/1
  BitwiseAND/1 -> [Byte_7_CAN1_DOA_Sta]
  bus_selector/2 -> [CAN1_EPB1_CS]  "<CAN1_EPB1_CS>"
  [CAN1_EPB1_CS] -> LeftShift1/1
  LeftShift1/1 -> BitwiseAND1/1
  BitwiseAND1/1 -> [Byte_0_CAN1_EPB1_CS]
  bus_selector/3 -> [CAN1_EPB1_RC]  "<CAN1_EPB1_RC>"
  [CAN1_EPB1_RC] -> LeftShift2/1
  LeftShift2/1 -> BitwiseAND2/1
  BitwiseAND2/1 -> [Byte_1_CAN1_EPB1_RC]
  bus_selector/4 -> [CAN1_EPBCarWashMode]  "<CAN1_EPBCarWashMode>"
  [CAN1_EPBCarWashMode] -> LeftShift3/1
  LeftShift3/1 -> BitwiseAND3/1
  BitwiseAND3/1 -> [Byte_7_CAN1_EPBCarWashMode]
  bus_selector/5 -> [CAN1_EPBErrSta]  "<CAN1_EPBErrSta>"
  [CAN1_EPBErrSta] -> LeftShift4/1
  LeftShift4/1 -> BitwiseAND4/1
  BitwiseAND4/1 -> [Byte_6_CAN1_EPBErrSta]
  bus_selector/6 -> [CAN1_EPBExtApplyAvail]  "<CAN1_EPBExtApplyAvail>"
  [CAN1_EPBExtApplyAvail] -> LeftShift5/1
  LeftShift5/1 -> BitwiseAND5/1
  BitwiseAND5/1 -> [Byte_7_CAN1_EPBExtApplyAvail]
  bus_selector/7 -> [CAN1_EPBExtReleaseAvail]  "<CAN1_EPBExtReleaseAvail>"
  [CAN1_EPBExtReleaseAvail] -> LeftShift6/1
  LeftShift6/1 -> BitwiseAND6/1
  BitwiseAND6/1 -> [Byte_7_CAN1_EPBExtReleaseAvail]
  bus_selector/8 -> [CAN1_EPBMsg]  "<CAN1_EPBMsg>"
  [CAN1_EPBMsg] -> LeftShift7/1
  LeftShift7/1 -> BitwiseAND7/1
  BitwiseAND7/1 -> [Byte_5_CAN1_EPBMsg]
  bus_selector/9 -> [CAN1_EPBRLampSta]  "<CAN1_EPBRLampSta>"
  [CAN1_EPBRLampSta] -> LeftShift8/1
  LeftShift8/1 -> BitwiseAND8/1
  BitwiseAND8/1 -> [Byte_6_CAN1_EPBRLampSta]
  bus_selector/10 -> [CAN1_EPBSta]  "<CAN1_EPBSta>"
  [CAN1_EPBSta] -> LeftShift9/1
  LeftShift9/1 -> BitwiseAND9/1
  BitwiseAND9/1 -> [Byte_5_CAN1_EPBSta]
  bus_selector/11 -> [CAN1_EPBStaL]  "<CAN1_EPBStaL>"
  [CAN1_EPBStaL] -> LeftShift10/1
  LeftShift10/1 -> BitwiseAND10/1
  BitwiseAND10/1 -> [Byte_7_CAN1_EPBStaL]
  bus_selector/12 -> [CAN1_EPBStaR]  "<CAN1_EPBStaR>"
  [CAN1_EPBStaR] -> LeftShift11/1
  LeftShift11/1 -> BitwiseAND11/1
  BitwiseAND11/1 -> [Byte_6_CAN1_EPBStaR]
  bus_selector/13 -> [CAN1_TakeOverReq]  "<CAN1_TakeOverReq>"
  [CAN1_TakeOverReq] -> LeftShift12/1
  LeftShift12/1 -> BitwiseAND12/1
  BitwiseAND12/1 -> [Byte_7_CAN1_TakeOverReq]
  Data Type Conversion/1 -> BitwiseOR/1
  [Byte_0_CAN1_EPB1_CS] -> Data Type Conversion/1
  BitwiseOR/1 -> [Byte_0]
  Data Type Conversion1/1 -> BitwiseOR1/1
  [Byte_1_CAN1_EPB1_RC] -> Data Type Conversion1/1
  BitwiseOR1/1 -> [Byte_1]
  constant/1 -> [Byte_2]
  constant1/1 -> [Byte_3]
  constant2/1 -> [Byte_4]
  Data Type Conversion2/1 -> BitwiseOR2/1
  [Byte_5_CAN1_EPBMsg] -> Data Type Conversion2/1
  Data Type Conversion3/1 -> BitwiseOR2/2
  [Byte_5_CAN1_EPBSta] -> Data Type Conversion3/1
  BitwiseOR2/1 -> [Byte_5]
  Data Type Conversion4/1 -> BitwiseOR3/1
  [Byte_6_CAN1_EPBErrSta] -> Data Type Conversion4/1
  Data Type Conversion5/1 -> BitwiseOR3/2
  [Byte_6_CAN1_EPBRLampSta] -> Data Type Conversion5/1
  Data Type Conversion6/1 -> BitwiseOR3/3
  [Byte_6_CAN1_EPBStaR] -> Data Type Conversion6/1
  BitwiseOR3/1 -> [Byte_6]
  Data Type Conversion7/1 -> BitwiseOR4/1
  [Byte_7_CAN1_DOA_Sta] -> Data Type Conversion7/1
  Data Type Conversion8/1 -> BitwiseOR4/2
  [Byte_7_CAN1_EPBCarWashMode] -> Data Type Conversion8/1
  Data Type Conversion9/1 -> BitwiseOR4/3
  [Byte_7_CAN1_EPBExtApplyAvail] -> Data Type Conversion9/1
  Data Type Conversion10/1 -> BitwiseOR4/4
  [Byte_7_CAN1_EPBExtReleaseAvail] -> Data Type Conversion10/1
  Data Type Conversion11/1 -> BitwiseOR4/5
  [Byte_7_CAN1_EPBStaL] -> Data Type Conversion11/1
  Data Type Conversion12/1 -> BitwiseOR4/6
  [Byte_7_CAN1_TakeOverReq] -> Data Type Conversion12/1
  BitwiseOR4/1 -> [Byte_7]
  [Byte_1] -> Mux/1
  [Byte_2] -> Mux/2
  [Byte_3] -> Mux/3
  [Byte_4] -> Mux/4
  [Byte_5] -> Mux/5
  [Byte_6] -> Mux/6
  [Byte_7] -> Mux/7
  Mux/1 -> [VHAL_CAN1EPB1noCS_raw]
  KHAL_CAN1EPB1E2E_flg/1 -> DDM_CS&RC_Comparison/1
  0x2B/1 -> DDM_CS&RC_Comparison/2
  0x7A/1 -> DDM_CS&RC_Comparison/3
  [VHAL_CAN1EPB1noCS_raw] -> DDM_CS&RC_Comparison/4
  [Byte_0] -> DDM_CS&RC_Comparison/5
  [RC_ECU] -> DDM_CS&RC_Comparison/6
  MessageRollingCounter/1 -> DDM_CS&RC_Comparison/7
  DDM_CS&RC_Comparison/1 -> VHAL_EPB1CSErr_flg/1
  DDM_CS&RC_Comparison/2 -> VHAL_EPB1RCErr_flg/1
  [DT_CAN1_SG_EPB1] -> bus_selector1/1
  bus_selector1/1 -> DOASta/1(DOA_Sta)  "<CAN1_DOA_Sta>"
  DOASta/1(VHAL_DOASta_flg) -> VHAL_DOASta_flg/1
  [DT_CAN1_SG_EPB1] -> bus_selector2/1
  bus_selector2/1 -> EPB1RC/1(EPB1_RC)  "<CAN1_EPB1_RC>"
  EPB1RC/1(VHAL_EPB1RC_enum) -> VHAL_EPB1RC_enum/1, [RC_ECU]
  [DT_CAN1_SG_EPB1] -> bus_selector3/1
  bus_selector3/1 -> EPBCarWashMode/1(EPBCarWashMode)  "<CAN1_EPBCarWashMode>"
  EPBCarWashMode/1(VHAL_EPBCarWashMode_flg) -> VHAL_EPBCarWashMode_flg/1
  [DT_CAN1_SG_EPB1] -> bus_selector4/1
  bus_selector4/1 -> EPBErrSta/1(EPBErrSta)  "<CAN1_EPBErrSta>"
  EPBErrSta/1(VHAL_EPBErrSta_enum) -> VHAL_EPBErrSta_enum/1
  [DT_CAN1_SG_EPB1] -> bus_selector5/1
  bus_selector5/1 -> EPBExtApplyAvail/1(EPBExtApplyAvail)  "<CAN1_EPBExtApplyAvail>"
  EPBExtApplyAvail/1(VHAL_EPBExtApplyAvail_flg) -> VHAL_EPBExtApplyAvail_flg/1
  [DT_CAN1_SG_EPB1] -> bus_selector6/1
  bus_selector6/1 -> EPBExtReleaseAvail/1(EPBExtReleaseAvail)  "<CAN1_EPBExtReleaseAvail>"
  EPBExtReleaseAvail/1(VHAL_EPBExtReleaseAvail_flg) -> VHAL_EPBExtReleaseAvail_flg/1
  [DT_CAN1_SG_EPB1] -> bus_selector7/1
  bus_selector7/1 -> EPBSta/1(EPBSta)  "<CAN1_EPBSta>"
  EPBSta/1(VHAL_EPBSta_enum) -> VHAL_EPBSta_enum/1
